simulink model "bitshiftandlogic"  (R2022b)
settings: Solver=VariableStepAuto  StartTime=0.0  StopTime=10.0  RelTol=1e-3
libraries: simulink x1
settings Model: Creator=Brigosha_Guest  LastModifiedBy=Brigosha_Guest

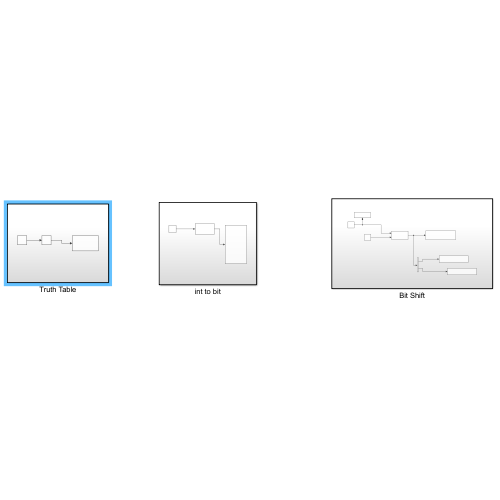
[thumbnail: Simulink's stored preview of the top-level diagram]
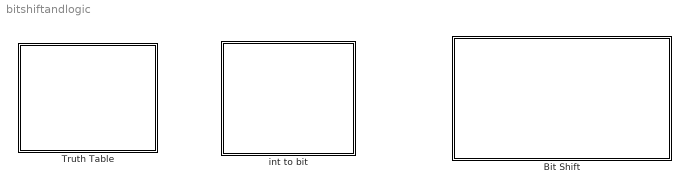
== system bitshiftandlogic ==
  Bit Shift : Subsystem
  Truth Table : Subsystem
  int to bit : Subsystem

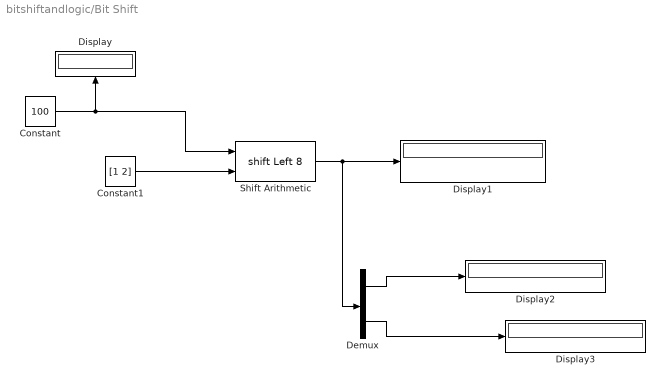
== system bitshiftandlogic/Bit Shift ==
  Constant : Constant  Value=100  OutDataTypeStr=int8
  Constant1 : Constant  Value=[1 2]  OutDataTypeStr=int8
  Demux : Demux  Outputs=2
  Display{,1..3} (4 alike) : Display
      settings: Format=binary (Stored Integer)
  Shift Arithmetic : ArithShift  BitShiftNumberSource=Input port  BitShiftNumber=8  BinPtShiftNumber=2  BitShiftDirection=Left  DiagnosticForOORShift=Warning
      settings: InputPortMap=u0,p1
  wires:
  Constant/1 -> Shift Arithmetic/1, Display/1
  Shift Arithmetic/1 -> Demux/1, Display1/1
  Demux/2 -> Display3/1
  Constant1/1 -> Shift Arithmetic/2
  Demux/1 -> Display2/1

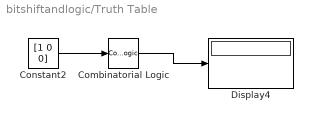
== system bitshiftandlogic/Truth Table ==
  Combinatorial Logic : CombinatorialLogic
  Constant2 : Constant  Value=[1 0 0]  OutDataTypeStr=boolean
  Display4 : Display
  wires:
  Combinatorial Logic/1 -> Display4/1
  Constant2/1 -> Combinatorial Logic/1

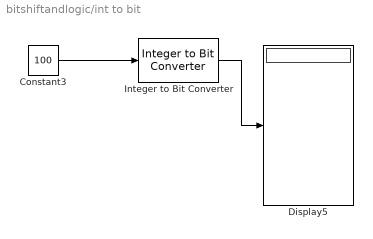
== system bitshiftandlogic/int to bit ==
  Constant3 : Constant  Value=100  OutDataTypeStr=int8
  Display5 : Display
  Integer to Bit Converter : simulink/Logic and Bit Operations/Integer to Bit Converter  nbits=8  signedInputValues=Signed  bitOrder=MSB first  outDtype=Inherit via internal rule
  wires:
  Constant3/1 -> Integer to Bit Converter/1
  Integer to Bit Converter/1 -> Display5/1
